simulink model "mod1"  (R2021b)
settings: Solver=FixedStepAuto  StartTime=0.0  StopTime=T_sim  FixedStep=Ts  RelTol=1e-3
values from neighbouring files (symbols this model uses):
  h1_ini = 0.7    [es1.m]    (also in exercise_session_1_classe.m)
  h1_ref = 1    [es1.m]    (also in exercise_session_1_classe.m)
  h2_ini = 0.6    [es1.m]    (also in exercise_session_1_classe.m)
  h2_ref = 1.2    [es1.m]    (also in exercise_session_1_classe.m)
  u1_max = 0.9    [es1.m]    (also in exercise_session_1_classe.m)
  u1_min = 0    [es1.m]    (also in exercise_session_1_classe.m)
  u1_ref = k*sqrt(h2_ref)    [es1.m]    (also in exercise_session_1_classe.m)
  u2_max = 0.9    [es1.m]    (also in exercise_session_1_classe.m)
  u2_min = 0    [es1.m]    (also in exercise_session_1_classe.m)
  u2_ref = u1_ref    [es1.m]    (also in exercise_session_1_classe.m)
libraries: cstblocks x3
settings Model: Creator=giuly  LastModifiedBy=giuly

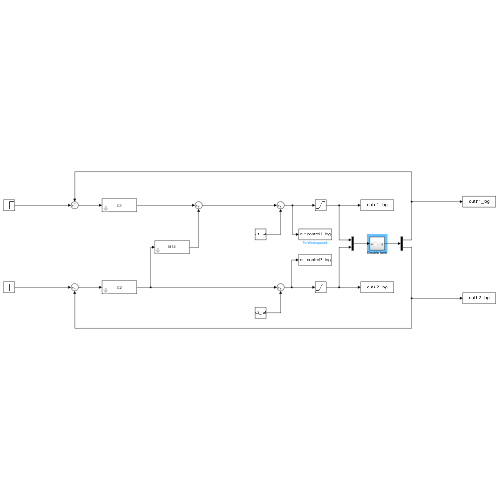
[thumbnail: Simulink's stored preview of the top-level diagram]
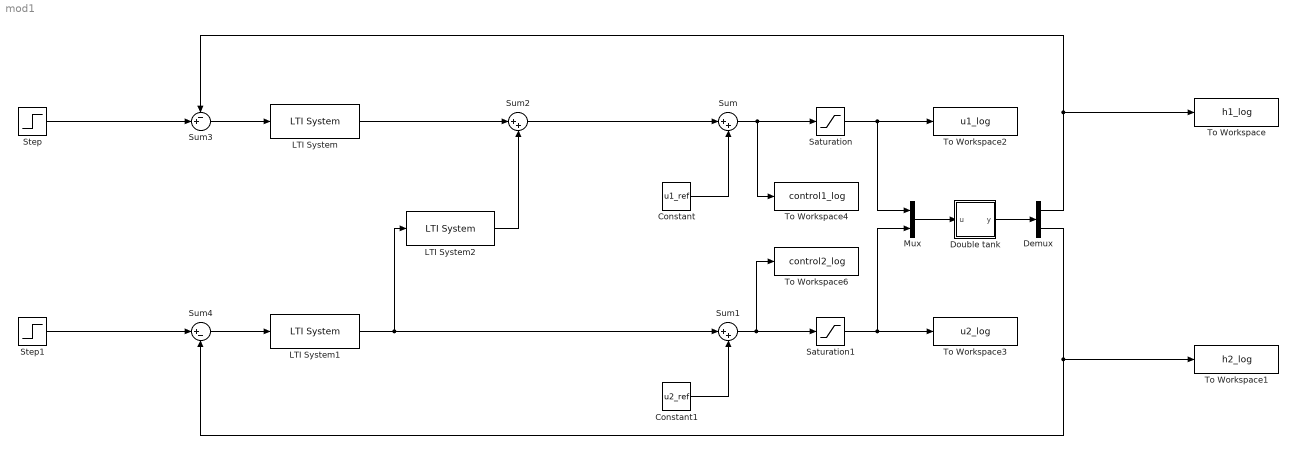
== system mod1 ==
  Constant : Constant  Value=u1_ref
  Constant1 : Constant  Value=u2_ref
  Demux : Demux  Outputs=2
  Double tank : Subsystem
  LTI System : cstblocks/LTI System  sys=C1  IC=[]
  LTI System1 : cstblocks/LTI System  sys=C2  IC=[]
  LTI System2 : cstblocks/LTI System  sys=M12  IC=[]
  Mux : Mux  Inputs=2
  Saturation : Saturate  UpperLimit=u1_max  LowerLimit=u1_min
  Saturation1 : Saturate  UpperLimit=u2_max  LowerLimit=u2_min
  Step : Step  Before=h1_ini  After=h1_ref  SampleTime=0
  Step1 : Step  Before=h2_ini  After=h2_ref  SampleTime=0
  Sum : Sum  Inputs=|++
  Sum1 : Sum  Inputs=|++
  Sum2 : Sum  Inputs=|++
  Sum3 : Sum  Inputs=-+|
  Sum4 : Sum  Inputs=|+-
  To Workspace : ToWorkspace  VariableName=h1_log  SaveFormat=Timeseries  SampleTime=-1
  To Workspace1 : ToWorkspace  VariableName=h2_log  SaveFormat=Timeseries  SampleTime=-1
  To Workspace2 : ToWorkspace  VariableName=u1_log  SaveFormat=Timeseries  SampleTime=-1
  To Workspace3 : ToWorkspace  VariableName=u2_log  SaveFormat=Timeseries  SampleTime=-1
  To Workspace4 : ToWorkspace  VariableName=control1_log  SaveFormat=Timeseries  SampleTime=-1
  To Workspace6 : ToWorkspace  VariableName=control2_log  SaveFormat=Timeseries  SampleTime=-1
  wires:
  Double tank/1(y) -> Demux/1
  Mux/1 -> Double tank/1(u)
  Saturation/1 -> To Workspace2/1, Mux/1
  Saturation1/1 -> Mux/2, To Workspace3/1
  Sum/1 -> To Workspace4/1, Saturation/1
  Sum1/1 -> Saturation1/1, To Workspace6/1
  Constant1/1 -> Sum1/2
  Constant/1 -> Sum/2
  LTI System/1 -> Sum2/1
  Sum2/1 -> Sum/1
  LTI System2/1 -> Sum2/2
  LTI System1/1 -> Sum1/1, LTI System2/1
  Demux/1 -> Sum3/1, To Workspace/1
  Sum3/1 -> LTI System/1
  Sum4/1 -> LTI System1/1
  Demux/2 -> Sum4/2, To Workspace1/1
  Step/1 -> Sum3/2
  Step1/1 -> Sum4/1

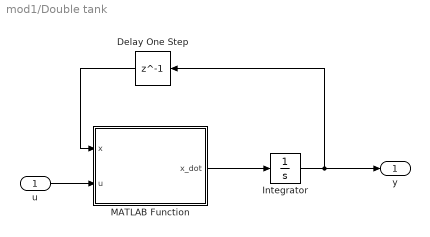
== system mod1/Double tank ==
  u : Inport
  Delay One Step : Delay  DelayLength=1  InitialCondition=[h1_ini; h2_ini]
  Integrator : Integrator  InitialCondition=[h1_ini; h2_ini]
  MATLAB Function : MATLAB Function  TreatAsAtomicUnit=on
  y : Outport
  wires:
  u/1 -> MATLAB Function/2(u)
  Integrator/1 -> y/1, Delay One Step/1
  Delay One Step/1 -> MATLAB Function/1(x)
  MATLAB Function/1(x_dot) -> Integrator/1

== matlab function mod1/Double tank/MATLAB Function ==
  data: x input; u input; x_dot output; k parameter
function x_dot = double_tank(x,u,k)

% Definizione iniziale del vettore x_dot
x_dot = zeros(2,1);

% Dinamica del sistema
x_dot(1) = u(1)-u(2);
x_dot(2) = u(2) - k*sqrt(x(2));
